simulink model "teleop_sampleddata_blocks2"  (R2019b)
settings: Solver=VariableStepAuto  StartTime=0.0  StopTime=20  RelTol=1e-3
values from neighbouring files (symbols this model uses):
  Be = 5    [normal_wave_architecture_constant_parameters.m]    (also in normal_wave_architecture_constant_parameters.m.m; normal_wave_architecture_variable_parameters.m)
  beta_m = 2*pi*Fc_vel*Ts    (= 0.0628318530718)    [normal_wave_architecture_constant_parameters.m]    (also in normal_wave_architecture_constant_parameters.m.m; normal_wave_architecture_variable_parameters.m)
  beta_s = 2*pi*Fc_vel*Ts    (= 0.0628318530718)    [normal_wave_architecture_constant_parameters.m]    (also in normal_wave_architecture_constant_parameters.m.m; normal_wave_architecture_variable_parameters.m)
  Bh = 0.02    [normal_wave_architecture_constant_parameters.m]    (also in normal_wave_architecture_constant_parameters.m.m; normal_wave_architecture_variable_parameters.m)
  d_m2s = 1    [normal_wave_architecture_constant_parameters.m]    (also in normal_wave_architecture_constant_parameters.m.m = 10; normal_wave_architecture_variable_parameters.m = 0.001)
  d_s2m = 1    [normal_wave_architecture_constant_parameters.m]    (also in normal_wave_architecture_constant_parameters.m.m = 10; normal_wave_architecture_variable_parameters.m = 0.001)
  eQ_m = 2*pi/4096    (= 0.00153398078789)    [normal_wave_architecture_constant_parameters.m]    (also in normal_wave_architecture_constant_parameters.m.m; normal_wave_architecture_variable_parameters.m)
  eQ_s = 2*pi/4096    (= 0.00153398078789)    [normal_wave_architecture_constant_parameters.m]    (also in normal_wave_architecture_constant_parameters.m.m; normal_wave_architecture_variable_parameters.m)
  Fc_h = 5    [normal_wave_architecture_constant_parameters.m]    (also in normal_wave_architecture_constant_parameters.m.m; normal_wave_architecture_variable_parameters.m)
  Jh = 0.02    [normal_wave_architecture_constant_parameters.m]    (also in normal_wave_architecture_constant_parameters.m.m; normal_wave_architecture_variable_parameters.m)
  k_m = 19.34    [normal_wave_architecture_constant_parameters.m]    (also in normal_wave_architecture_constant_parameters.m.m; normal_wave_architecture_variable_parameters.m)
  k_s = 19.34    [normal_wave_architecture_constant_parameters.m]    (also in normal_wave_architecture_constant_parameters.m.m; normal_wave_architecture_variable_parameters.m)
  Kc2v_m = 4.5    [normal_wave_architecture_constant_parameters.m]    (also in normal_wave_architecture_constant_parameters.m.m; normal_wave_architecture_variable_parameters.m)
  Kc2v_s = 4.5    [normal_wave_architecture_constant_parameters.m]    (also in normal_wave_architecture_constant_parameters.m.m; normal_wave_architecture_variable_parameters.m)
  Kd_h = 0.5    [normal_wave_architecture_constant_parameters.m]    (also in normal_wave_architecture_constant_parameters.m.m; normal_wave_architecture_variable_parameters.m)
  Kd_m = 0.5    [normal_wave_architecture_constant_parameters.m]    (also in normal_wave_architecture_constant_parameters.m.m; normal_wave_architecture_variable_parameters.m)
  Kd_s = 0.5    [normal_wave_architecture_constant_parameters.m]    (also in normal_wave_architecture_constant_parameters.m.m; normal_wave_architecture_variable_parameters.m)
  Ke = 10    [normal_wave_architecture_constant_parameters.m]    (also in normal_wave_architecture_constant_parameters.m.m; normal_wave_architecture_variable_parameters.m)
  Kp_h = 1.2    [normal_wave_architecture_constant_parameters.m]    (also in normal_wave_architecture_constant_parameters.m.m; normal_wave_architecture_variable_parameters.m)
  Kp_m = 1    [normal_wave_architecture_constant_parameters.m]    (also in normal_wave_architecture_constant_parameters.m.m; normal_wave_architecture_variable_parameters.m)
  Kp_s = 1    [normal_wave_architecture_constant_parameters.m]    (also in normal_wave_architecture_constant_parameters.m.m; normal_wave_architecture_variable_parameters.m)
  Kt2c_m = 1.182    [normal_wave_architecture_constant_parameters.m]    (also in normal_wave_architecture_constant_parameters.m.m; normal_wave_architecture_variable_parameters.m)
  Kt2c_s = 1.182    [normal_wave_architecture_constant_parameters.m]    (also in normal_wave_architecture_constant_parameters.m.m; normal_wave_architecture_variable_parameters.m)
  lArm_m = 0.1    [normal_wave_architecture_constant_parameters.m]    (also in normal_wave_architecture_constant_parameters.m.m; normal_wave_architecture_variable_parameters.m)
  lArm_s = 0.1    [normal_wave_architecture_constant_parameters.m]    (also in normal_wave_architecture_constant_parameters.m.m; normal_wave_architecture_variable_parameters.m)
  qe = 0.5    [normal_wave_architecture_constant_parameters.m]    (also in normal_wave_architecture_constant_parameters.m.m; normal_wave_architecture_variable_parameters.m)
  tau_m = 1.217    [normal_wave_architecture_constant_parameters.m]    (also in normal_wave_architecture_constant_parameters.m.m; normal_wave_architecture_variable_parameters.m)
  tau_s = 1.217    [normal_wave_architecture_constant_parameters.m]    (also in normal_wave_architecture_constant_parameters.m.m; normal_wave_architecture_variable_parameters.m)
  Ts = 0.001    [normal_wave_architecture_constant_parameters.m]    (also in normal_wave_architecture_constant_parameters.m.m; normal_wave_architecture_variable_parameters.m; wave_s.m = Is)
libraries: simulink x2
settings Model: Creator=riccardo  LastModifiedBy=luigi

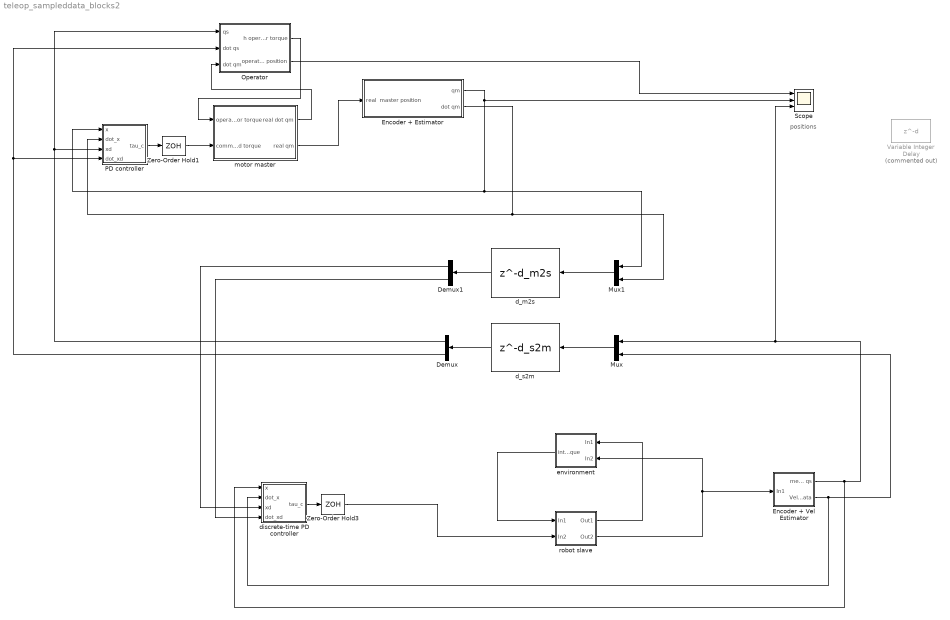
== system teleop_sampleddata_blocks2 ==
  note: positions
  Demux : Demux  Outputs=2
  Demux1 : Demux  Outputs=2
  Encoder + Estimator : Subsystem
  "Encoder + Vel Estimator " : Subsystem
  Mux : Mux  Inputs=2
  Mux1 : Mux  Inputs=2
  Operator : Subsystem
  PD controller : Subsystem
  Scope : Scope  NumInputPorts=3
  Variable Integer Delay : Delay  Commented=on  DelayLengthSource=Input port
      settings: InputPortMap=u0,p1
  Zero-Order Hold1 : ZeroOrderHold  SampleTime=Ts
  Zero-Order Hold3 : ZeroOrderHold  SampleTime=Ts
  "d_m2s " : Delay  DelayLength=d_m2s  SampleTime=Ts
  "d_s2m " : Delay  DelayLength=d_s2m  SampleTime=Ts
  discrete-time PD controller : Subsystem
  "environment " : Subsystem
  motor master : Subsystem
  "robot slave " : Subsystem
  wires:
  discrete-time PD controller/1(tau_c) -> Zero-Order Hold3/1
  "robot slave "/2(Out2) -> "environment "/2(In2), "Encoder + Vel Estimator "/1(In1)
  Zero-Order Hold3/1 -> "robot slave "/2(In2)
  "robot slave "/1(Out1) -> "environment "/1(In1)
  "environment "/1("interaction torque ") -> "robot slave "/1(In1)
  "Encoder + Vel Estimator "/1("meas qs ") -> Scope/3, Mux/1, discrete-time PD controller/1(x)
  "Encoder + Vel Estimator "/2("Vel Stimata ") -> Mux/2, discrete-time PD controller/2(dot_x)
  Encoder + Estimator/1(qm) -> Scope/2, PD controller/1(x), Mux1/1
  Operator/1(h operator torque) -> motor master/1(operator torque)
  PD controller/1(tau_c) -> Zero-Order Hold1/1
  motor master/2(real qm) -> Encoder + Estimator/1(real  master position)
  Demux/2 -> Operator/2(dot qs), PD controller/4(dot_xd)
  motor master/1(real dot qm) -> Operator/3(dot qm)
  Zero-Order Hold1/1 -> motor master/2(command torque)
  Demux/1 -> Operator/1(qs), PD controller/3(xd)
  Encoder + Estimator/2(dot qm) -> PD controller/2(dot_x), Mux1/2
  Mux/1 -> "d_s2m "/1
  "d_s2m "/1 -> Demux/1
  "d_m2s "/1 -> Demux1/1
  Mux1/1 -> "d_m2s "/1
  Demux1/1 -> discrete-time PD controller/3(xd)
  Demux1/2 -> discrete-time PD controller/4(dot_xd)
  Operator/2("operator position ") -> Scope/1

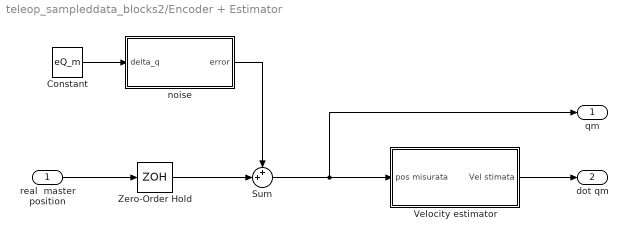
== system teleop_sampleddata_blocks2/Encoder + Estimator ==
  real  master position : Inport
  Constant : Constant  Value=eQ_m
  Sum : Sum  Inputs=++|
  Velocity estimator : Subsystem
  Zero-Order Hold : ZeroOrderHold  SampleTime=Ts
  noise : MATLAB Function  TreatAsAtomicUnit=on
  qm : Outport
  dot qm : Outport  Port=2
  wires:
  real  master position/1 -> Zero-Order Hold/1
  Zero-Order Hold/1 -> Sum/2
  Sum/1 -> qm/1, Velocity estimator/1(pos misurata)
  Constant/1 -> noise/1(delta_q)
  Velocity estimator/1(Vel stimata) -> dot qm/1
  noise/1(error) -> Sum/1

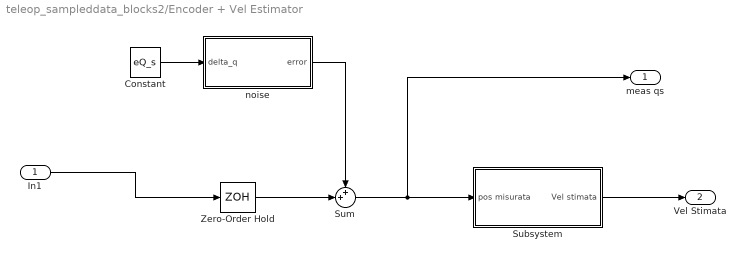
== system teleop_sampleddata_blocks2/Encoder + Vel Estimator  ==
  In1 : Inport
  Constant : Constant  Value=eQ_s
  Subsystem : Subsystem
  Sum : Sum  Inputs=++|
  Zero-Order Hold : ZeroOrderHold  SampleTime=Ts
  noise : MATLAB Function  TreatAsAtomicUnit=on
  "meas qs " : Outport
  "Vel Stimata " : Outport  Port=2
  wires:
  Constant/1 -> noise/1(delta_q)
  In1/1 -> Zero-Order Hold/1
  noise/1(error) -> Sum/1
  Zero-Order Hold/1 -> Sum/2
  Sum/1 -> "meas qs "/1, Subsystem/1(pos misurata)
  Subsystem/1(Vel stimata) -> "Vel Stimata "/1

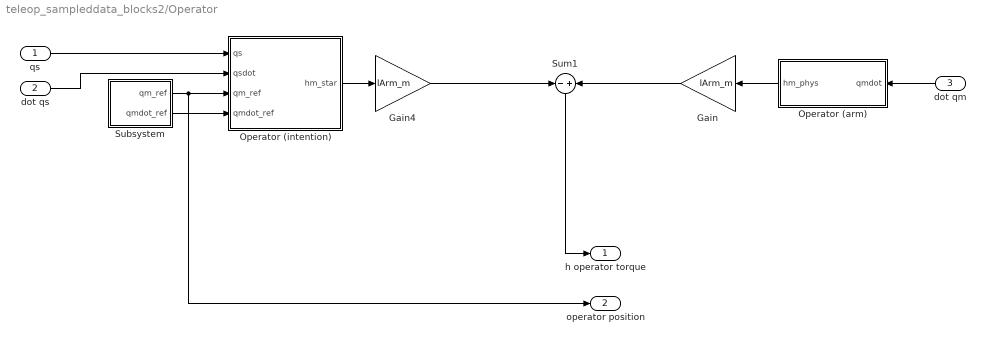
== system teleop_sampleddata_blocks2/Operator ==
  qs : Inport
  dot qs : Inport  Port=2
  dot qm : Inport  Port=3
  Gain : Gain  Gain=lArm_m
  Gain4 : Gain  Gain=lArm_m
  Operator (arm) : Subsystem
  Operator (intention) : Subsystem
  Subsystem : Subsystem
  Sum1 : Sum  Inputs=-+
  h operator torque : Outport
  "operator position " : Outport  Port=2
  wires:
  Sum1/1 -> h operator torque/1
  Operator (arm)/1(hm_phys) -> Gain/1
  dot qm/1 -> Operator (arm)/1(qmdot)
  Subsystem/2(qmdot_ref) -> Operator (intention)/4(qmdot_ref)
  Operator (intention)/1(hm_star) -> Gain4/1
  dot qs/1 -> Operator (intention)/2(qsdot)
  Gain4/1 -> Sum1/1
  Gain/1 -> Sum1/2
  Subsystem/1(qm_ref) -> "operator position "/1, Operator (intention)/3(qm_ref)
  qs/1 -> Operator (intention)/1(qs)

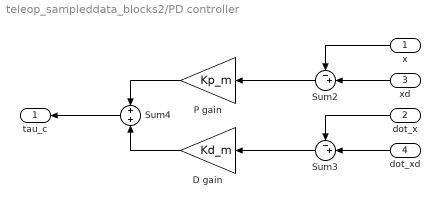
== system teleop_sampleddata_blocks2/PD controller ==
  x : Inport
  dot_x : Inport  Port=2
  xd : Inport  Port=3
  dot_xd : Inport  Port=4
  D gain : Gain  Gain=Kd_m
  P gain : Gain  Gain=Kp_m
  Sum2 : Sum  Inputs=-+|
  Sum3 : Sum  Inputs=-+|
  Sum4 : Sum
  tau_c : Outport  VectorParamsAs1DForOutWhenUnconnected=off
  wires:
  D gain/1 -> Sum4/2
  dot_x/1 -> Sum3/1
  dot_xd/1 -> Sum3/2
  x/1 -> Sum2/1
  xd/1 -> Sum2/2
  Sum3/1 -> D gain/1
  P gain/1 -> Sum4/1
  Sum4/1 -> tau_c/1
  Sum2/1 -> P gain/1

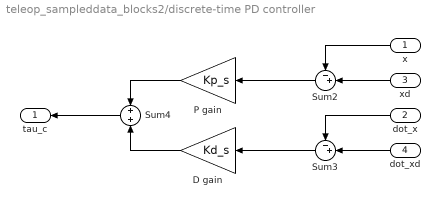
== system teleop_sampleddata_blocks2/discrete-time PD controller ==
  x : Inport
  dot_x : Inport  Port=2
  xd : Inport  Port=3
  dot_xd : Inport  Port=4
  D gain : Gain  Gain=Kd_s
  P gain : Gain  Gain=Kp_s
  Sum2 : Sum  Inputs=-+|
  Sum3 : Sum  Inputs=-+|
  Sum4 : Sum
  tau_c : Outport  VectorParamsAs1DForOutWhenUnconnected=off
  wires:
  D gain/1 -> Sum4/2
  dot_x/1 -> Sum3/1
  dot_xd/1 -> Sum3/2
  x/1 -> Sum2/1
  xd/1 -> Sum2/2
  Sum3/1 -> D gain/1
  P gain/1 -> Sum4/1
  Sum4/1 -> tau_c/1
  Sum2/1 -> P gain/1

== system teleop_sampleddata_blocks2/environment  ==
  note: qs
  note: qdot
  In1 : Inport
  In2 : Inport  Port=2
  Environment : Subsystem
  Gain : Gain  Gain=lArm_s
  "interaction torque " : Outport
  wires:
  In2/1 -> Environment/2(qs)
  Environment/1(fe) -> Gain/1
  In1/1 -> Environment/1(qsdot)
  Gain/1 -> "interaction torque "/1

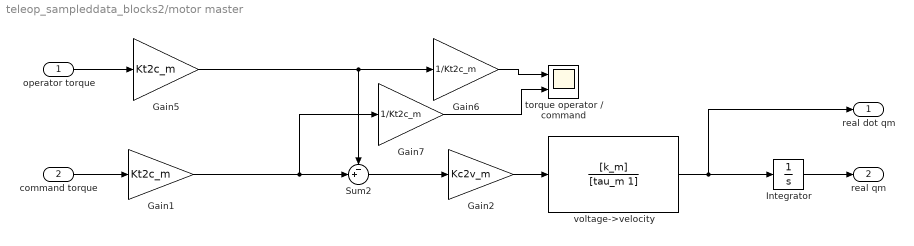
== system teleop_sampleddata_blocks2/motor master ==
  operator torque : Inport
  command torque : Inport  Port=2
  Gain1 : Gain  Gain=Kt2c_m
  Gain2 : Gain  Gain=Kc2v_m
  Gain5 : Gain  Gain=Kt2c_m
  Gain6 : Gain  Gain=1/Kt2c_m
  Gain7 : Gain  Gain=1/Kt2c_m
  Integrator : Integrator
  Sum2 : Sum  Inputs=-+|
  torque operator / command : Scope  NumInputPorts=2
  voltage->velocity : TransferFcn  Numerator=[k_m]  Denominator=[tau_m 1]
  real dot qm : Outport
  real qm : Outport  Port=2
  wires:
  Gain7/1 -> torque operator / command/2
  operator torque/1 -> Gain5/1
  Gain2/1 -> voltage->velocity/1
  Gain1/1 -> Gain7/1, Sum2/2
  Integrator/1 -> real qm/1
  command torque/1 -> Gain1/1
  Gain6/1 -> torque operator / command/1
  voltage->velocity/1 -> real dot qm/1, Integrator/1
  Sum2/1 -> Gain2/1
  Gain5/1 -> Sum2/1, Gain6/1

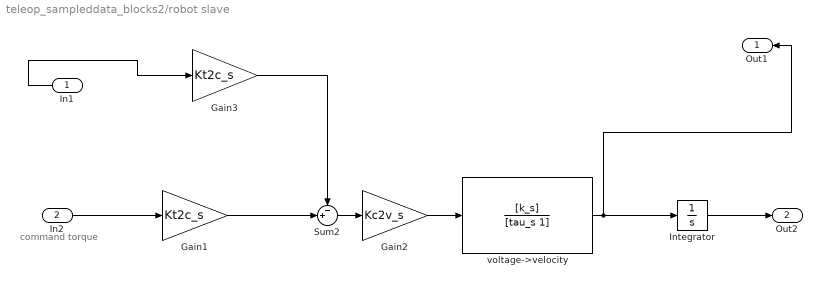
== system teleop_sampleddata_blocks2/robot slave  ==
  note: command torque
  In1 : Inport
  In2 : Inport  Port=2
  Gain1 : Gain  Gain=Kt2c_s
  Gain2 : Gain  Gain=Kc2v_s
  Gain3 : Gain  Gain=Kt2c_s
  Integrator : Integrator
  Sum2 : Sum  Inputs=-+|
  voltage->velocity : TransferFcn  Numerator=[k_s]  Denominator=[tau_s 1]
  Out1 : Outport
  Out2 : Outport  Port=2
  wires:
  Gain2/1 -> voltage->velocity/1
  Gain3/1 -> Sum2/1
  voltage->velocity/1 -> Out1/1, Integrator/1
  Gain1/1 -> Sum2/2
  Sum2/1 -> Gain2/1
  Integrator/1 -> Out2/1
  In1/1 -> Gain3/1
  In2/1 -> Gain1/1

== system teleop_sampleddata_blocks2/Encoder + Estimator/Velocity estimator ==
  pos misurata : Inport
  Difference : simulink/Discrete/Difference  ICPrevInput=0.0  OutMin=[]  OutMax=[]  OutDataType=fixdt(1, 16)  OutScaling=2^-10  DoSatur=off
  Filtro passabasso : DiscreteTransferFcn  Numerator=[beta_m 0]  Denominator=[1 -(1-beta_m)]  SampleTime=Ts
  Gain2 : Gain  Gain=1/Ts
  Vel stimata : Outport  VectorParamsAs1DForOutWhenUnconnected=off
  wires:
  Gain2/1 -> Filtro passabasso/1
  pos misurata/1 -> Difference/1
  Difference/1 -> Gain2/1
  Filtro passabasso/1 -> Vel stimata/1  "Velocità  stimata"

== system teleop_sampleddata_blocks2/Encoder + Vel Estimator /Subsystem ==
  pos misurata : Inport
  Difference : simulink/Discrete/Difference  ICPrevInput=0.0  OutMin=[]  OutMax=[]  OutDataType=fixdt(1, 16)  OutScaling=2^-10  DoSatur=off
  Filtro passabasso : DiscreteTransferFcn  Numerator=[beta_s 0]  Denominator=[1 -(1-beta_s)]  SampleTime=Ts
  Gain2 : Gain  Gain=1/Ts
  Vel stimata : Outport  VectorParamsAs1DForOutWhenUnconnected=off
  wires:
  Gain2/1 -> Filtro passabasso/1
  pos misurata/1 -> Difference/1
  Difference/1 -> Gain2/1
  Filtro passabasso/1 -> Vel stimata/1  "Velocità  stimata"

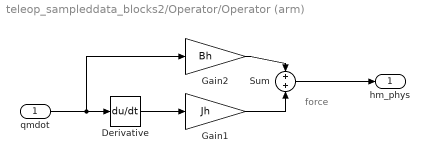
== system teleop_sampleddata_blocks2/Operator/Operator (arm) ==
  note: force
  qmdot : Inport
  Derivative : Derivative  CoefficientInTFapproximation=0.001
  Gain1 : Gain  Gain=Jh
  Gain2 : Gain  Gain=Bh
  Sum : Sum  Inputs=+|+
  hm_phys : Outport  VectorParamsAs1DForOutWhenUnconnected=off
  wires:
  qmdot/1 -> Gain2/1, Derivative/1
  Sum/1 -> hm_phys/1
  Derivative/1 -> Gain1/1
  Gain2/1 -> Sum/1
  Gain1/1 -> Sum/2

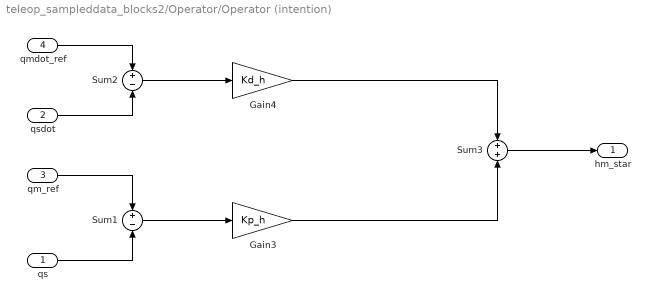
== system teleop_sampleddata_blocks2/Operator/Operator (intention) ==
  qs : Inport
  qsdot : Inport  Port=2
  qm_ref : Inport  Port=3
  qmdot_ref : Inport  Port=4
  Gain3 : Gain  Gain=Kp_h
  Gain4 : Gain  Gain=Kd_h
  Sum1 : Sum  Inputs=+|-
  Sum2 : Sum  Inputs=+|-
  Sum3 : Sum  Inputs=+|+
  hm_star : Outport  VectorParamsAs1DForOutWhenUnconnected=off
  wires:
  qs/1 -> Sum1/2
  qm_ref/1 -> Sum1/1
  qmdot_ref/1 -> Sum2/1
  Sum1/1 -> Gain3/1
  qsdot/1 -> Sum2/2
  Sum2/1 -> Gain4/1
  Gain4/1 -> Sum3/1
  Gain3/1 -> Sum3/2
  Sum3/1 -> hm_star/1

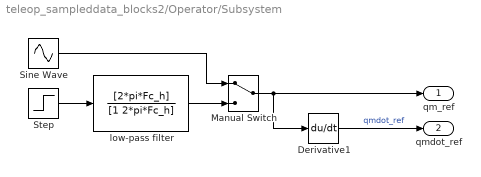
== system teleop_sampleddata_blocks2/Operator/Subsystem ==
  Derivative1 : Derivative  CoefficientInTFapproximation=0.001
  Manual Switch : ManualSwitch
  Sine Wave : Sin  SampleTime=0
  Step : Step  SampleTime=0
  low-pass filter : TransferFcn  Numerator=[2*pi*Fc_h]  Denominator=[1 2*pi*Fc_h]
  qm_ref : Outport
  qmdot_ref : Outport  Port=2
  wires:
  low-pass filter/1 -> Manual Switch/2
  Manual Switch/1 -> qm_ref/1, Derivative1/1
  Derivative1/1 -> qmdot_ref/1  "qmdot_ref"
  Step/1 -> low-pass filter/1
  Sine Wave/1 -> Manual Switch/1

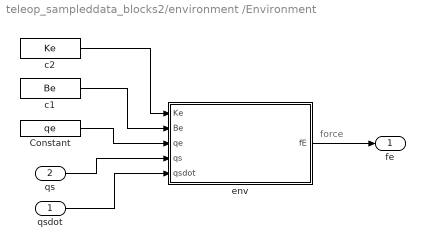
== system teleop_sampleddata_blocks2/environment /Environment ==
  note: force
  qsdot : Inport
  qs : Inport  Port=2
  Constant : Constant  Value=qe  SampleTime=0
  c1 : Constant  Value=Be  SampleTime=0
  c2 : Constant  Value=Ke  SampleTime=0
  env : MATLAB Function  TreatAsAtomicUnit=on
  fe : Outport  VectorParamsAs1DForOutWhenUnconnected=off
  wires:
  Constant/1 -> env/3(qe)
  c1/1 -> env/2(Be)
  c2/1 -> env/1(Ke)
  qs/1 -> env/4(qs)
  qsdot/1 -> env/5(qsdot)
  env/1(fE) -> fe/1

== matlab function teleop_sampleddata_blocks2/Encoder + Vel Estimator /noise ==
  data: delta_q input; error output
function error = noise_measurement(delta_q)
if randn(1)>0
   error = delta_q;
else
    error = -delta_q;
end

== matlab function teleop_sampleddata_blocks2/Encoder + Estimator/noise ==
  data: delta_q input; error output
function error = noise_measurement(delta_q)
if randn(1)>0
   error = delta_q;
else
    error = -delta_q;
end

== matlab function teleop_sampleddata_blocks2/environment /Environment/env ==
  data: Ke input; Be input; qe input; qs input; fE output; qsdot input
function fE  = environment(Ke, Be, qe, qs, qsdot)
if qs > qe
   fE = Ke * (qs - qe) + Be * qsdot;
else
   fE = 0;
end
